simulink model "MIL4L3_SW6_V1_20220211"  (R2018b)
settings: Solver=FixedStepAuto  StartTime=0.0  StopTime=inf  FixedStep=0.001  RelTol=1e-3
PreLoadFcn:
  | A0_MILtest;
undefined symbols (not defined in the file or in its folder): Clb_ICADirect_LaneDisp_StateFive, Clb_ICADirect_LaneDisp_StateFour, Clb_ICADirect_LaneDisp_StateOne, Clb_ICADirect_LaneDisp_StateThree, Clb_ICADirect_LaneDisp_StateTwo, Clb_ICADirect_LaneDisp_StateZero, Clb_ICADirect_LaneDispSW, Clb_ICADirect_TrnLghtsCom_Switch, Clb_ICADirect_TrnLghtsCom_Value, Clb_ICADirect_TrnLghtsCrtl_Inhb, IMAP_Clb_ACU_Driver_Belt, IMAP_Clb_ACU_Driver_Belt_Over, IMAP_Clb_ACU_Passenger_Belt, IMAP_Clb_ACU_Passenger_Belt_Over, IMAP_Clb_ACU_RearLeft_Belt, IMAP_Clb_ACU_RearLeft_Belt_Over, IMAP_Clb_ACU_RearMiddle_Belt, IMAP_Clb_ACU_RearMiddle_Belt_Over, IMAP_Clb_ACU_RearRight_Belt, IMAP_Clb_ACU_RearRight_Belt_Over, IMAP_Clb_AEB_Switch, IMAP_Clb_AEB_Switch_Over, IMAP_Clb_ALC_TLC_Mode, IMAP_Clb_ALC_TLC_Mode_Over, IMAP_Clb_BCM_Battery_Voltage, IMAP_Clb_BCM_Battery_Voltage_Over, IMAP_Clb_BCM_BrakeLamp_State, IMAP_Clb_BCM_BrakeLamp_State_Over, IMAP_Clb_BCM_CHMSL_Status, IMAP_Clb_BCM_CHMSL_Status_Over, IMAP_Clb_BCM_Door_Lock_State, IMAP_Clb_BCM_Door_Lock_State_Over, IMAP_Clb_BCM_FrontWiper_State, IMAP_Clb_BCM_FrontWiper_State_Over, IMAP_Clb_BCM_FrontWiper_Switch, IMAP_Clb_BCM_FrontWiper_Switch_Over, IMAP_Clb_BCM_HazardLamp, IMAP_Clb_BCM_HazardLamp_Over, IMAP_Clb_BCM_HazardLamp_Switch, IMAP_Clb_BCM_HazardLamp_Switch_Over, IMAP_Clb_BCM_HighBeam_State, IMAP_Clb_BCM_HighBeam_State_Over, IMAP_Clb_BCM_Ignition_State, IMAP_Clb_BCM_Ignition_State_Over, IMAP_Clb_BCM_IHBC_Enabled, IMAP_Clb_BCM_IHBC_Enabled_Over, IMAP_Clb_BCM_Left_Light, IMAP_Clb_BCM_Left_Light_Over, IMAP_Clb_BCM_LeftTurn_Switch, IMAP_Clb_BCM_LeftTurn_Switch_Over, IMAP_Clb_BCM_LF_Door_State, IMAP_Clb_BCM_LF_Door_State_Over, IMAP_Clb_BCM_LowBeam_State, IMAP_Clb_BCM_LowBeam_State_Over, IMAP_Clb_BCM_LR_Door_State, IMAP_Clb_BCM_LR_Door_State_Over, IMAP_Clb_BCM_RF_Door_State, IMAP_Clb_BCM_RF_Door_State_Over, IMAP_Clb_BCM_Right_Light, IMAP_Clb_BCM_Right_Light_Over ... (+547)
libraries: CarMaker4SL x2153, simulink x292, dspstat3 x3, canmsglib x2, simulink_extras x1
(part 8 of 52)

== system MIL4L3_SW6_V1_20220211/CarMaker/VehicleControl/Function/ACC ==
  Bus Selector : BusSelector  OutputSignals=IMAPve_d_ISA_Switch,IMAPve_d_ISA_ISLC_Mode,IMAPve_d_Speed_Limit,IMAPve_d_ALC_TLC_Mode,IMAPve_d_EPS_LKA_State,IMAPve_g_EPS_SW_Trq,IMAPve_d_EPS_Trq_State,IMAPve_d_SAS_Clb_State,IMAPve_d_SAS_Trim_State,IMAPve_d_EPS_TrqLim_State,IMAPve_g_EPS_LKA_Current,IMAPve_g_ESC_LatAcc,IMAPve_d_ESC_LatAcc_Valid,IMAPve_g_ESC_YawRate,IMAPve_d_ESC_YawRate_Valid,IMAPve_g_ESC_UnYawRate,IMAPve_g_ESC_VehSpd,IMAPve_g_ESC_LonAcc,IMAPve_d_ESC_LonAcc_Valid,IMAPve_g_ESC_Brake_Press,IMAPve_g_ESC_Static_Slope,IMAPve_g_ESC_DySlope_Accuracy,IMAPve_g_ESC_DySlope,IMAPve_g_SW_Angle,IMAPve_g_SW_Angle_Speed,IMAPve_d_BCM_HazardLamp,IMAPve_d_BCM_Left_Light,IMAPve_d_BCM_Right_Light,IMAPve_d_ESC_BrakeLamp_Req,IMAPve_d_BCM_Opening_State,IMAPve_d_BCM_Trunk_State,IMAPve_d_BCM_LF_Door_State,IMAPve_d_BCM_RF_Door_State,IMAPve_d_BCM_RR_Door_State,IMAPve_d_BCM_LR_Door_State,IMAPve_d_SCC_Left_SwitchSig,IMAPve_d_SCC_Right_SwitchSig,IMAPve_d_EMS_ACC_Status,IMAPve_g_EMS_Pot_WhlT_Max,IMAPve_g_EMS_Pot_WhlT_Min,IMAPve_g_EMS_RealPedal,IMAPve_g_EMS_MaxTWhl,IMAPve_g_EMS_MaxTWhl_Offset,IMAPve_g_EMS_MinTWhl,IMAPve_g_EMS_MinTWhl_Offset,IMAPve_g_EMS_Actual_FlwT,IMAPve_g_EMS_Actual_IndT,IMAPve_g_EMS_Realize_TWhl,IMAPve_g_EMS_ACC_VirtualPedal,IMAPve_d_EMS_AccPedal_Fault,IMAPve_g_EMS_Driver_Torque,IMAPve_d_ESC_Brake_Effort,IMAPve_g_EMS_Engine_Speed,IMAPve_d_ESC_Veh_Standstill,IMAPve_d_TCU_Actual_Gear,IMAPve_d_TCU_Target_Gear,IMAPve_d_TCU_PRND_State,IMAPve_d_BCM_Ignition_State,IMAPve_d_ACU_Driver_Belt,IMAPve_d_SWS_Failure_Status,IMAPve_d_ESC_OFF,IMAPve_d_ESC_AlarmSig,IMAPve_d_ESC_ESC_Active,IMAPve_d_ESC_MSR_Active,IMAPve_d_ESC_TCS_Active,IMAPve_d_ESC_VehSpd_Valid,IMAPve_d_ESC_ABS_Active,IMAPve_d_ESC_ABS_Valid,IMAPve_d_ESC_ABS_AlarmSig,IMAPve_d_ESC_FL_WheelPulVal,IMAPve_d_ESC_FR_WheelPulVal,IMAPve_d_ESC_RL_WheelPulVal,IMAPve_d_ESC_RR_WheelPulVal,IMAPve_g_ESC_FL_WhlSpd,IMAPve_d_ESC_FL_WhlSpd_Fault,IMAPve_g_ESC_FR_WhlSpd,IMAPve_d_ESC_FR_WhlSpd_Fault,IMAPve_g_ESC_RL_WhlSpd,IMAPve_d_ESC_RL_WhlSpd_Fault,IMAPve_g_ESC_RR_WhlSpd,IMAPve_d_ESC_RR_WhlSpd_Fault,IMAPve_d_ESC_FL_Wheel_Pulse,IMAPve_d_ESC_FR_Wheel_Pulse,IMAPve_d_ESC_RL_Wheel_Pulse,IMAPve_d_ESC_RR_Wheel_Pulse,IMAPve_d_TCU_AT_Failure,IMAPve_d_TCU_Shift_Valid,IMAPve_d_TCU_DCT_Clutch_State,IMAPve_d_TCU_Gear_Engage,IMAPve_d_TCU_Select_ATMode,IMAPve_d_EMS_Engine_Status,IMAPve_d_EMS_Gearbox_CtlAvail,IMAPve_d_ESC_Brake_Failsafe,IMAPve_d_ESC_ACC_Available,IMAPve_d_ESC_ACC_Active,IMAPve_d_EMS_ACC_Effective,IMAPve_d_BCM_FrontWiper_State,IMAPve_d_BCM_CHMSL_Status,IMAPve_d_BCM_BrakeLamp_State,IMAPve_d_ACU_Passenger_Belt,IMAPve_d_EMS_ACC_CtlAvail,IMAPve_d_EMS_ACC_Inhibited,IMAPve_d_EMS_Brake_Pedal,IMAPve_d_BCM_LowBeam_State,IMAPve_d_BCM_HighBeam_State,IMAPve_d_EPB_Status,IMAPve_d_ESC_Drive_Direction,IMAPve_d_ESC_Hold_State,IMAPve_d_EPS_Steer_Hold_State,IMAPve_d_EPS_Warning_State,IMAPve_g_EPS_PowerCon,IMAPve_d_ESC_EBD_AlarmSig,IMAPve_d_ESC_AVH_Status,IMAPve_d_Radar_State,IMAPve_d_Time_System_Clock
  Bus Selector1 : BusSelector  OutputSignals=IMAPve_d_ORI_CIPV_ID,IMAPve_d_ORI_Obj_Num,IMAPva_d_ORI_Obj_Class,IMAPva_g_ORI_Obj_RelVel,IMAPva_g_ORI_Obj_LongDis,IMAPva_g_ORI_Obj_LAngle,IMAPva_g_ORI_Obj_RAngle,IMAPva_g_ORI_Obj_Width,IMAPva_d_ORI_Obj_ID,IMAPve_g_ORI_L0_C3,IMAPve_g_ORI_L0_C2,IMAPve_g_ORI_L0_C1,IMAPve_g_ORI_L0_C0,IMAPve_d_ORI_L0_Type,IMAPve_g_ORI_L0_VR,IMAPve_g_ORI_L0_W,IMAPve_g_ORI_L1_C3,IMAPve_g_ORI_L1_C2,IMAPve_g_ORI_L1_C1,IMAPve_g_ORI_L1_C0,IMAPve_d_ORI_L1_Type,IMAPve_g_ORI_L1_VR,IMAPve_g_ORI_L1_W,IMAPve_g_ORI_R0_C3,IMAPve_g_ORI_R0_C2,IMAPve_g_ORI_R0_C1,IMAPve_g_ORI_R0_C0,IMAPve_d_ORI_R0_LT,IMAPve_g_ORI_R0_VR,IMAPve_g_ORI_R0_W,IMAPve_g_ORI_R1_C3,IMAPve_g_ORI_R1_C2,IMAPve_g_ORI_R1_C1,IMAPve_g_ORI_R1_C0,IMAPve_d_ORI_R1_LT,IMAPve_g_ORI_R1_VR,IMAPve_g_ORI_R1_W,IMAPve_d_Sensor_Status,IMAPve_d_LF_Radar_Status,IMAPve_d_RF_Radar_Status,IMAPve_d_LR_Radar_Status,IMAPve_d_RR_Radar_Status,IMAPve_d_Fusion_Status,IMAPve_d_Fusion_Time_Stamp,IMAPve_d_obj_Num,IMAPva_d_obj_id,IMAPva_g_obj_pos_x,IMAPva_g_obj_pos_y,IMAPva_g_obj_vel_x,IMAPva_g_obj_vel_y,IMAPva_g_obj_acc_x,IMAPva_g_obj_acc_y,IMAPva_g_obj_pos_var_x,IMAPva_g_obj_pos_var_y,IMAPva_g_obj_pos_var_xy,IMAPva_g_obj_width,IMAPva_g_obj_length,IMAPva_d_obj_class,IMAPva_d_obj_lane,IMAPva_d_obj_status,IMAPva_d_obj_age,IMAPva_d_obj_TurnLight,IMAPva_d_obj_BrakeLight,IMAPva_d_obj_MotionStatus,IMAPve_d_Road_Type,IMAPve_g_L0_C0,IMAPve_g_L0_C1,IMAPve_g_L0_C2,IMAPve_g_L0_C3,IMAPve_g_L0_VR,IMAPve_d_L0_Q,IMAPve_d_L0_Type,IMAPve_g_L0_W,IMAPve_g_R0_C0,IMAPve_g_R0_C1,IMAPve_g_R0_C2,IMAPve_g_R0_C3,IMAPve_g_R0_VR,IMAPve_d_R0_Q,IMAPve_d_R0_Type,IMAPve_g_R0_W,IMAPve_g_L1_C0,IMAPve_g_L1_C1,IMAPve_g_L1_C2,IMAPve_g_L1_C3,IMAPve_g_L1_VR,IMAPve_d_L1_Q,IMAPve_d_L1_Type,IMAPve_g_L1_W,IMAPve_g_R1_C0,IMAPve_g_R1_C1,IMAPve_g_R1_C2,IMAPve_g_R1_C3,IMAPve_g_R1_VR,IMAPve_d_R1_Q,IMAPve_d_R1_Type,IMAPve_g_R1_W,IMAPve_g_L0_C0_Back,IMAPve_g_L0_C1_Back,IMAPve_g_L0_C2_Back,IMAPve_g_L0_C3_Back,IMAPve_g_L0_Range_Back,IMAPve_g_R0_C0_Back,IMAPve_g_R0_C1_Back,IMAPve_g_R0_C2_Back,IMAPve_g_R0_C3_Back,IMAPve_g_R0_Range_Back,IMAPve_g_L1_C0_Back,IMAPve_g_L1_C1_Back,IMAPve_g_L1_C2_Back,IMAPve_g_L1_C3_Back,IMAPve_g_L1_Range_Back,IMAPve_g_R1_C0_Back,IMAPve_g_R1_C1_Back,IMAPve_g_R1_C2_Back,IMAPve_g_R1_C3_Back,IMAPve_g_R1_Range_Back,IMAPve_d_Sign_ISA_Value,IMAPve_g_Camera_Signal_Fault,IMAPve_d_Camera_State,IMAPve_d_ESC_FLW_Direction,IMAPve_d_ESC_FRW_Direction,IMAPve_d_ESC_TCS_ErrorStatus,IMAPve_d_ESC_RLW_Direction,IMAPve_d_ESC_RRW_Direction,IMAPve_d_ESC_EPB_ErrorStatus,IMAPve_d_EPS_SteeringAngle_Flag,IMAPve_g_EPS_SteeringAngle,IMAPve_d_EPS_Driver_Override,IMAPve_d_EPS_Driver_Active_ESA,IMAPve_d_EPS_ESA_State,IMAPve_d_ACU_RearLeft_Belt,IMAPve_d_ACU_RearMiddle_Belt,IMAPve_d_ACU_RearRight_Belt,IMAPve_d_EMS_PowertrainCtl_State,IMAPve_d_TCU_TCU_Available,IMAPve_d_BCM_LeftTurn_Switch,IMAPve_d_BCM_RightTurn_Switch,IMAPve_d_MP5_AutoPilot_Switch,IMAPve_d_MP5_DMS_Sensity,IMAPve_d_MP5_DMS_EyeFatigue,IMAPve_d_MP5_DMS_LongtimeDrive,IMAPve_d_MP5_DMS_SideView,IMAPve_d_MP5_DMS_UsingPhone,IMAPve_d_MP5_DMS_Smoking,IMAPve_d_MP5_DMS_DrinkWater,IMAPve_d_APA_AutoPark_WorkSt,IMAPve_g_ESC_BrkWhlCylinder_Pressure,IMAPve_d_ISA_Status,IMAPve_d_ISA_Sign_Type,IMAPve_d_ISA_Popup_Message
  Bus Selector2 : BusSelector  OutputSignals=IMAPve_d_Camera_State
  Bus Selector3 : BusSelector  OutputSignals=AEBSve_d_AEBAlertReq
  Bus Selector4 : BusSelector  OutputSignals=IMAPva_g_ORI_Obj_ExistProb,IMAPve_d_Radar_FaultBitSetting_Signal
  Bus Selector5 : BusSelector  OutputSignals=IMAPve_d_BCM_HazardLamp_Switch
  BusCreator : BusCreator  Inputs=27
  Clock : Clock
  Data Type Conversion{,1..11,13,23..24} (15 alike) : DataTypeConversion
  Delay : Delay  DelayLength=1
  Model1 : ModelReference  ModelNameDialog=ACCS_SW6_20220127_Version.slxp  ModelReferenceVersion=1.4  CopyOfModelProtected=on
  tag scope: ACCSva_d_ACCS2ICAB=global, ACC_output=global, ADAS_ACC_State=global
  wires:
  Clock/1 -> Data Type Conversion/1  "TIME_System_Clock"
  Model1/1 -> [ADAS_ACC_State], BusCreator/1  "ACCSve_d_ACC_State"
  Model1/2 -> BusCreator/2  "ACCSve_g_ACC_TqReq"
  Model1/3 -> BusCreator/3  "ACCSve_d_ACC_TqFlag"
  Model1/4 -> BusCreator/4  "ACCSve_g_ACC_DecReq"
  Model1/5 -> BusCreator/5  "ACCSve_d_ACC_DecFlag"
  Model1/6 -> BusCreator/6  "ACCSve_d_CIPV_ID"
  Model1/7 -> BusCreator/7  "ACCSve_d_ACCActive_Signal"
  Model1/8 -> BusCreator/8  "ACCSve_d_ACC_go_request"
  Model1/9 -> BusCreator/9  "ACCSve_d_VelocitySet"
  Model1/10 -> BusCreator/10  "ACCSve_d_HeadWaySet"
  Model1/11 -> Delay/1, BusCreator/11  "ACCSva_d_ACCS2ICA"
  [ICABva_d_ICAB2ACCS] -> Model1/119
  [FDMMve_d_AccFcnConf] -> Model1/118
  Delay/1 -> [ACCSva_d_ACCS2ICAB]
  Data Type Conversion23/1 -> BusCreator/14  "ACCSve_d_ACC_ESCDriverOff"
  Data Type Conversion24/1 -> BusCreator/15  "ACCSve_d_ACC_ESCHoldReq"
  Data Type Conversion1/1 -> BusCreator/16  "ACCSve_d_ACC_EPBReq"
  Model1/16 -> Data Type Conversion1/1
  Model1/15 -> Data Type Conversion24/1
  Model1/14 -> Data Type Conversion23/1
  Data Type Conversion/1 -> Model1/116
  BusCreator/1 -> [ACC_output]
  Model1/17 -> Data Type Conversion2/1
  Model1/18 -> Data Type Conversion3/1
  Model1/19 -> Data Type Conversion4/1
  Model1/20 -> Data Type Conversion5/1
  Model1/21 -> Data Type Conversion6/1
  Model1/22 -> Data Type Conversion8/1
  Model1/23 -> Data Type Conversion7/1
  Model1/24 -> Data Type Conversion9/1
  Model1/25 -> Data Type Conversion10/1
  Model1/26 -> Data Type Conversion11/1
  Data Type Conversion2/1 -> BusCreator/17  "ACCSve_d_ACC_ISLCState"
  Data Type Conversion3/1 -> BusCreator/18  "ACCSve_d_ACC_ISLCDriverRemind"
  Data Type Conversion4/1 -> BusCreator/19  "ACCSve_d_ACCMessagePrompt"
  Data Type Conversion5/1 -> BusCreator/20  "ACCSve_g_ob1H_10"
  Data Type Conversion6/1 -> BusCreator/21  "ACCSve_g_ob1L_10"
  Data Type Conversion8/1 -> BusCreator/22  "ACCSve_g_ob2H_10"
  Data Type Conversion7/1 -> BusCreator/23  "ACCSve_g_ob2L_10"
  Data Type Conversion9/1 -> BusCreator/24  "ACCSve_g_ob01H_100"
  Data Type Conversion10/1 -> BusCreator/25  "ACCSve_g_ob01L_100"
  Data Type Conversion11/1 -> BusCreator/26  "ACCSve_g_ob02H_100"
  [AEBSve_d_MDDdecRequest] -> Model1/117
  Model1/12 -> BusCreator/12  "ACCSve_d_SignalTStamp"
  Model1/13 -> BusCreator/13  "ACCSve_d_ACC_ICA_Flag"
  Model1/27 -> Data Type Conversion13/1  "ACCSve_g_ob02L_100"
  Data Type Conversion13/1 -> BusCreator/27  "ACCSve_g_ob02L_100"
  [IMAP_Output] -> Bus Selector5/1, Bus Selector4/1, Bus Selector2/1, Bus Selector1/1, Bus Selector/1
  Bus Selector/5 -> Model1/5  "<IMAPve_d_EPS_LKA_State>"
  [AEB_output] -> Bus Selector3/1
  Bus Selector3/1 -> Model1/271  "<AEBSve_d_AEBAlertReq>"
  Bus Selector2/1 -> Model1/272  "<IMAPve_d_Camera_State>"
  Bus Selector/1 -> Model1/1  "<IMAPve_d_ISA_Switch>"
  Bus Selector/2 -> Model1/2  "<IMAPve_d_ISA_ISLC_Mode>"
  Bus Selector/3 -> Model1/3  "<IMAPve_d_Speed_Limit>"
  Bus Selector/4 -> Model1/4  "<IMAPve_d_ALC_TLC_Mode>"
  Bus Selector/6 -> Model1/6  "<IMAPve_g_EPS_SW_Trq>"
  Bus Selector/7 -> Model1/7  "<IMAPve_d_EPS_Trq_State>"
  Bus Selector/8 -> Model1/8  "<IMAPve_d_SAS_Clb_State>"
  Bus Selector/9 -> Model1/9  "<IMAPve_d_SAS_Trim_State>"
  Bus Selector/10 -> Model1/10  "<IMAPve_d_EPS_TrqLim_State>"
  Bus Selector/11 -> Model1/11  "<IMAPve_g_EPS_LKA_Current>"
  Bus Selector/12 -> Model1/12  "<IMAPve_g_ESC_LatAcc>"
  Bus Selector/13 -> Model1/13  "<IMAPve_d_ESC_LatAcc_Valid>"
  Bus Selector/14 -> Model1/14  "<IMAPve_g_ESC_YawRate>"
  Bus Selector/15 -> Model1/15  "<IMAPve_d_ESC_YawRate_Valid>"
  Bus Selector/16 -> Model1/16  "<IMAPve_g_ESC_UnYawRate>"
  Bus Selector/17 -> Model1/17  "<IMAPve_g_ESC_VehSpd>"
  Bus Selector/18 -> Model1/18  "<IMAPve_g_ESC_LonAcc>"
  Bus Selector/19 -> Model1/19  "<IMAPve_d_ESC_LonAcc_Valid>"
  Bus Selector/20 -> Model1/20  "<IMAPve_g_ESC_Brake_Press>"
  Bus Selector/21 -> Model1/21  "<IMAPve_g_ESC_Static_Slope>"
  Bus Selector/22 -> Model1/22  "<IMAPve_g_ESC_DySlope_Accuracy>"
  Bus Selector/23 -> Model1/23  "<IMAPve_g_ESC_DySlope>"
  Bus Selector/24 -> Model1/24  "<IMAPve_g_SW_Angle>"
  Bus Selector/25 -> Model1/25  "<IMAPve_g_SW_Angle_Speed>"
  Bus Selector/26 -> Model1/26  "<IMAPve_d_BCM_HazardLamp>"
  Bus Selector/27 -> Model1/27  "<IMAPve_d_BCM_Left_Light>"
  Bus Selector/28 -> Model1/28  "<IMAPve_d_BCM_Right_Light>"
  Bus Selector/29 -> Model1/29  "<IMAPve_d_ESC_BrakeLamp_Req>"
  Bus Selector/30 -> Model1/30  "<IMAPve_d_BCM_Opening_State>"
  Bus Selector/31 -> Model1/31  "<IMAPve_d_BCM_Trunk_State>"
  Bus Selector/32 -> Model1/32  "<IMAPve_d_BCM_LF_Door_State>"
  Bus Selector/33 -> Model1/33  "<IMAPve_d_BCM_RF_Door_State>"
  Bus Selector/34 -> Model1/34  "<IMAPve_d_BCM_RR_Door_State>"
  Bus Selector/35 -> Model1/35  "<IMAPve_d_BCM_LR_Door_State>"
  Bus Selector/36 -> Model1/36  "<IMAPve_d_SCC_Left_SwitchSig>"
  Bus Selector/37 -> Model1/37  "<IMAPve_d_SCC_Right_SwitchSig>"
  Bus Selector/38 -> Model1/38  "<IMAPve_d_EMS_ACC_Status>"
  Bus Selector/39 -> Model1/39  "<IMAPve_g_EMS_Pot_WhlT_Max>"
  Bus Selector/40 -> Model1/40  "<IMAPve_g_EMS_Pot_WhlT_Min>"
  Bus Selector/41 -> Model1/41  "<IMAPve_g_EMS_RealPedal>"
  Bus Selector/42 -> Model1/42  "<IMAPve_g_EMS_MaxTWhl>"
  Bus Selector/43 -> Model1/43  "<IMAPve_g_EMS_MaxTWhl_Offset>"
  Bus Selector/44 -> Model1/44  "<IMAPve_g_EMS_MinTWhl>"
  Bus Selector/45 -> Model1/45  "<IMAPve_g_EMS_MinTWhl_Offset>"
  Bus Selector/46 -> Model1/46  "<IMAPve_g_EMS_Actual_FlwT>"
  Bus Selector/47 -> Model1/47  "<IMAPve_g_EMS_Actual_IndT>"
  Bus Selector/48 -> Model1/48  "<IMAPve_g_EMS_Realize_TWhl>"
  Bus Selector/49 -> Model1/49  "<IMAPve_g_EMS_ACC_VirtualPedal>"
  Bus Selector/50 -> Model1/50  "<IMAPve_d_EMS_AccPedal_Fault>"
  Bus Selector/51 -> Model1/51  "<IMAPve_g_EMS_Driver_Torque>"
  Bus Selector/52 -> Model1/52  "<IMAPve_d_ESC_Brake_Effort>"
  Bus Selector/53 -> Model1/53  "<IMAPve_g_EMS_Engine_Speed>"
  Bus Selector/54 -> Model1/54  "<IMAPve_d_ESC_Veh_Standstill>"
  Bus Selector/55 -> Model1/55  "<IMAPve_d_TCU_Actual_Gear>"
  Bus Selector/56 -> Model1/56  "<IMAPve_d_TCU_Target_Gear>"
  Bus Selector/57 -> Model1/57  "<IMAPve_d_TCU_PRND_State>"
  Bus Selector/58 -> Model1/58  "<IMAPve_d_BCM_Ignition_State>"
  Bus Selector/59 -> Model1/59  "<IMAPve_d_ACU_Driver_Belt>"
  Bus Selector/60 -> Model1/60  "<IMAPve_d_SWS_Failure_Status>"
  Bus Selector/61 -> Model1/61  "<IMAPve_d_ESC_OFF>"
  Bus Selector/62 -> Model1/62  "<IMAPve_d_ESC_AlarmSig>"
  Bus Selector/63 -> Model1/63  "<IMAPve_d_ESC_ESC_Active>"
  Bus Selector/64 -> Model1/64  "<IMAPve_d_ESC_MSR_Active>"
  Bus Selector/65 -> Model1/65  "<IMAPve_d_ESC_TCS_Active>"
  Bus Selector/66 -> Model1/66  "<IMAPve_d_ESC_VehSpd_Valid>"
  Bus Selector/67 -> Model1/67  "<IMAPve_d_ESC_ABS_Active>"
  Bus Selector/68 -> Model1/68  "<IMAPve_d_ESC_ABS_Valid>"
  Bus Selector/69 -> Model1/69  "<IMAPve_d_ESC_ABS_AlarmSig>"
  Bus Selector/70 -> Model1/70  "<IMAPve_d_ESC_FL_WheelPulVal>"
  Bus Selector/71 -> Model1/71  "<IMAPve_d_ESC_FR_WheelPulVal>"
  Bus Selector/72 -> Model1/72  "<IMAPve_d_ESC_RL_WheelPulVal>"
  Bus Selector/73 -> Model1/73  "<IMAPve_d_ESC_RR_WheelPulVal>"
  Bus Selector/74 -> Model1/74  "<IMAPve_g_ESC_FL_WhlSpd>"
  Bus Selector/75 -> Model1/75  "<IMAPve_d_ESC_FL_WhlSpd_Fault>"
  Bus Selector/76 -> Model1/76  "<IMAPve_g_ESC_FR_WhlSpd>"
  Bus Selector/77 -> Model1/77  "<IMAPve_d_ESC_FR_WhlSpd_Fault>"
  Bus Selector/78 -> Model1/78  "<IMAPve_g_ESC_RL_WhlSpd>"
  Bus Selector/79 -> Model1/79  "<IMAPve_d_ESC_RL_WhlSpd_Fault>"
  Bus Selector/80 -> Model1/80  "<IMAPve_g_ESC_RR_WhlSpd>"
  Bus Selector/81 -> Model1/81  "<IMAPve_d_ESC_RR_WhlSpd_Fault>"
  Bus Selector/82 -> Model1/82  "<IMAPve_d_ESC_FL_Wheel_Pulse>"
  Bus Selector/83 -> Model1/83  "<IMAPve_d_ESC_FR_Wheel_Pulse>"
  Bus Selector/84 -> Model1/84  "<IMAPve_d_ESC_RL_Wheel_Pulse>"
  Bus Selector/85 -> Model1/85  "<IMAPve_d_ESC_RR_Wheel_Pulse>"
  Bus Selector/86 -> Model1/86  "<IMAPve_d_TCU_AT_Failure>"
  Bus Selector/87 -> Model1/87  "<IMAPve_d_TCU_Shift_Valid>"
  Bus Selector/88 -> Model1/88  "<IMAPve_d_TCU_DCT_Clutch_State>"
  Bus Selector/89 -> Model1/89  "<IMAPve_d_TCU_Gear_Engage>"
  Bus Selector/90 -> Model1/90  "<IMAPve_d_TCU_Select_ATMode>"
  Bus Selector/91 -> Model1/91  "<IMAPve_d_EMS_Engine_Status>"
  Bus Selector/92 -> Model1/92  "<IMAPve_d_EMS_Gearbox_CtlAvail>"
  Bus Selector/93 -> Model1/93  "<IMAPve_d_ESC_Brake_Failsafe>"
  Bus Selector/94 -> Model1/94  "<IMAPve_d_ESC_ACC_Available>"
  Bus Selector/95 -> Model1/95  "<IMAPve_d_ESC_ACC_Active>"
  Bus Selector/96 -> Model1/96  "<IMAPve_d_EMS_ACC_Effective>"
  Bus Selector/97 -> Model1/97  "<IMAPve_d_BCM_FrontWiper_State>"
  Bus Selector/98 -> Model1/98  "<IMAPve_d_BCM_CHMSL_Status>"
  Bus Selector/99 -> Model1/99  "<IMAPve_d_BCM_BrakeLamp_State>"
  Bus Selector/100 -> Model1/100  "<IMAPve_d_ACU_Passenger_Belt>"
  Bus Selector/101 -> Model1/101  "<IMAPve_d_EMS_ACC_CtlAvail>"
  Bus Selector/102 -> Model1/102  "<IMAPve_d_EMS_ACC_Inhibited>"
  Bus Selector/103 -> Model1/103  "<IMAPve_d_EMS_Brake_Pedal>"
  Bus Selector/104 -> Model1/104  "<IMAPve_d_BCM_LowBeam_State>"
  Bus Selector/105 -> Model1/105  "<IMAPve_d_BCM_HighBeam_State>"
  Bus Selector/106 -> Model1/106  "<IMAPve_d_EPB_Status>"
  Bus Selector/107 -> Model1/107  "<IMAPve_d_ESC_Drive_Direction>"
  Bus Selector/108 -> Model1/108  "<IMAPve_d_ESC_Hold_State>"
  Bus Selector/109 -> Model1/109  "<IMAPve_d_EPS_Steer_Hold_State>"
  Bus Selector/110 -> Model1/110  "<IMAPve_d_EPS_Warning_State>"
  Bus Selector/111 -> Model1/111  "<IMAPve_g_EPS_PowerCon>"
  Bus Selector/112 -> Model1/112  "<IMAPve_d_ESC_EBD_AlarmSig>"
  Bus Selector/113 -> Model1/113  "<IMAPve_d_ESC_AVH_Status>"
  Bus Selector/114 -> Model1/114  "<IMAPve_d_Radar_State>"
  Bus Selector/115 -> Model1/115  "<IMAPve_d_Time_System_Clock>"
  Bus Selector1/1 -> Model1/120  "<IMAPve_d_ORI_CIPV_ID>"
  Bus Selector1/2 -> Model1/121  "<IMAPve_d_ORI_Obj_Num>"
  Bus Selector1/3 -> Model1/122  "<IMAPva_d_ORI_Obj_Class>"
  Bus Selector1/4 -> Model1/123  "<IMAPva_g_ORI_Obj_RelVel>"
  Bus Selector1/5 -> Model1/124  "<IMAPva_g_ORI_Obj_LongDis>"
  Bus Selector1/6 -> Model1/125  "<IMAPva_g_ORI_Obj_LAngle>"
  Bus Selector1/7 -> Model1/126  "<IMAPva_g_ORI_Obj_RAngle>"
  Bus Selector1/8 -> Model1/127  "<IMAPva_g_ORI_Obj_Width>"
  Bus Selector1/9 -> Model1/128  "<IMAPva_d_ORI_Obj_ID>"
  Bus Selector1/10 -> Model1/129  "<IMAPve_g_ORI_L0_C3>"
  Bus Selector1/11 -> Model1/130  "<IMAPve_g_ORI_L0_C2>"
  Bus Selector1/12 -> Model1/131  "<IMAPve_g_ORI_L0_C1>"
  Bus Selector1/13 -> Model1/132  "<IMAPve_g_ORI_L0_C0>"
  Bus Selector1/14 -> Model1/133  "<IMAPve_d_ORI_L0_Type>"
  Bus Selector1/15 -> Model1/134  "<IMAPve_g_ORI_L0_VR>"
  Bus Selector1/16 -> Model1/135  "<IMAPve_g_ORI_L0_W>"
  Bus Selector1/17 -> Model1/136  "<IMAPve_g_ORI_L1_C3>"
  Bus Selector1/18 -> Model1/137  "<IMAPve_g_ORI_L1_C2>"
  Bus Selector1/19 -> Model1/138  "<IMAPve_g_ORI_L1_C1>"
  Bus Selector1/20 -> Model1/139  "<IMAPve_g_ORI_L1_C0>"
  Bus Selector1/21 -> Model1/140  "<IMAPve_d_ORI_L1_Type>"
  Bus Selector1/22 -> Model1/141  "<IMAPve_g_ORI_L1_VR>"
  Bus Selector1/23 -> Model1/142  "<IMAPve_g_ORI_L1_W>"
  Bus Selector1/24 -> Model1/143  "<IMAPve_g_ORI_R0_C3>"
  Bus Selector1/25 -> Model1/144  "<IMAPve_g_ORI_R0_C2>"
  Bus Selector1/26 -> Model1/145  "<IMAPve_g_ORI_R0_C1>"
  Bus Selector1/27 -> Model1/146  "<IMAPve_g_ORI_R0_C0>"
  Bus Selector1/28 -> Model1/147  "<IMAPve_d_ORI_R0_LT>"
  Bus Selector1/29 -> Model1/148  "<IMAPve_g_ORI_R0_VR>"
  Bus Selector1/30 -> Model1/149  "<IMAPve_g_ORI_R0_W>"
  Bus Selector1/31 -> Model1/150  "<IMAPve_g_ORI_R1_C3>"
  Bus Selector1/32 -> Model1/151  "<IMAPve_g_ORI_R1_C2>"
  Bus Selector1/33 -> Model1/152  "<IMAPve_g_ORI_R1_C1>"
  Bus Selector1/34 -> Model1/153  "<IMAPve_g_ORI_R1_C0>"
  Bus Selector1/35 -> Model1/154  "<IMAPve_d_ORI_R1_LT>"
  Bus Selector1/36 -> Model1/155  "<IMAPve_g_ORI_R1_VR>"
  Bus Selector1/37 -> Model1/156  "<IMAPve_g_ORI_R1_W>"
  Bus Selector1/38 -> Model1/157  "<IMAPve_d_Sensor_Status>"
  Bus Selector1/39 -> Model1/158  "<IMAPve_d_LF_Radar_Status>"
  Bus Selector1/40 -> Model1/159  "<IMAPve_d_RF_Radar_Status>"
  Bus Selector1/41 -> Model1/160  "<IMAPve_d_LR_Radar_Status>"
  Bus Selector1/42 -> Model1/161  "<IMAPve_d_RR_Radar_Status>"
  Bus Selector1/43 -> Model1/162  "<IMAPve_d_Fusion_Status>"
  Bus Selector1/44 -> Model1/163  "<IMAPve_d_Fusion_Time_Stamp>"
  Bus Selector1/45 -> Model1/164  "<IMAPve_d_obj_Num>"
  Bus Selector1/46 -> Model1/165  "<IMAPva_d_obj_id>"
  Bus Selector1/47 -> Model1/166  "<IMAPva_g_obj_pos_x>"
  Bus Selector1/48 -> Model1/167  "<IMAPva_g_obj_pos_y>"
  Bus Selector1/49 -> Model1/168  "<IMAPva_g_obj_vel_x>"
  Bus Selector1/50 -> Model1/169  "<IMAPva_g_obj_vel_y>"
  Bus Selector1/51 -> Model1/170  "<IMAPva_g_obj_acc_x>"
  Bus Selector1/52 -> Model1/171  "<IMAPva_g_obj_acc_y>"
  Bus Selector1/53 -> Model1/172  "<IMAPva_g_obj_pos_var_x>"
  Bus Selector1/54 -> Model1/173  "<IMAPva_g_obj_pos_var_y>"
  Bus Selector1/55 -> Model1/174  "<IMAPva_g_obj_pos_var_xy>"
  Bus Selector1/56 -> Model1/175  "<IMAPva_g_obj_width>"
  Bus Selector1/57 -> Model1/176  "<IMAPva_g_obj_length>"
  Bus Selector1/58 -> Model1/177  "<IMAPva_d_obj_class>"
  Bus Selector1/59 -> Model1/178  "<IMAPva_d_obj_lane>"
  Bus Selector1/60 -> Model1/179  "<IMAPva_d_obj_status>"
  Bus Selector1/61 -> Model1/180  "<IMAPva_d_obj_age>"
  Bus Selector1/62 -> Model1/181  "<IMAPva_d_obj_TurnLight>"
  Bus Selector1/63 -> Model1/182  "<IMAPva_d_obj_BrakeLight>"
  Bus Selector1/64 -> Model1/183  "<IMAPva_d_obj_MotionStatus>"
  Bus Selector1/65 -> Model1/184  "<IMAPve_d_Road_Type>"
  Bus Selector1/66 -> Model1/185  "<IMAPve_g_L0_C0>"
  Bus Selector1/67 -> Model1/186  "<IMAPve_g_L0_C1>"
  Bus Selector1/68 -> Model1/187  "<IMAPve_g_L0_C2>"
  Bus Selector1/69 -> Model1/188  "<IMAPve_g_L0_C3>"
  Bus Selector1/70 -> Model1/189  "<IMAPve_g_L0_VR>"
  Bus Selector1/71 -> Model1/190  "<IMAPve_d_L0_Q>"
  Bus Selector1/72 -> Model1/191  "<IMAPve_d_L0_Type>"
  Bus Selector1/73 -> Model1/192  "<IMAPve_g_L0_W>"
  Bus Selector1/74 -> Model1/193  "<IMAPve_g_R0_C0>"
  Bus Selector1/75 -> Model1/194  "<IMAPve_g_R0_C1>"
  Bus Selector1/76 -> Model1/195  "<IMAPve_g_R0_C2>"
  Bus Selector1/77 -> Model1/196  "<IMAPve_g_R0_C3>"
  Bus Selector1/78 -> Model1/197  "<IMAPve_g_R0_VR>"
  Bus Selector1/79 -> Model1/198  "<IMAPve_d_R0_Q>"
  Bus Selector1/80 -> Model1/199  "<IMAPve_d_R0_Type>"
  Bus Selector1/81 -> Model1/200  "<IMAPve_g_R0_W>"
  Bus Selector1/82 -> Model1/201  "<IMAPve_g_L1_C0>"
  Bus Selector1/83 -> Model1/202  "<IMAPve_g_L1_C1>"
  Bus Selector1/84 -> Model1/203  "<IMAPve_g_L1_C2>"
  Bus Selector1/85 -> Model1/204  "<IMAPve_g_L1_C3>"
  Bus Selector1/86 -> Model1/205  "<IMAPve_g_L1_VR>"
  Bus Selector1/87 -> Model1/206  "<IMAPve_d_L1_Q>"
  Bus Selector1/88 -> Model1/207  "<IMAPve_d_L1_Type>"
  Bus Selector1/89 -> Model1/208  "<IMAPve_g_L1_W>"
  Bus Selector1/90 -> Model1/209  "<IMAPve_g_R1_C0>"
  Bus Selector1/91 -> Model1/210  "<IMAPve_g_R1_C1>"
  Bus Selector1/92 -> Model1/211  "<IMAPve_g_R1_C2>"
  Bus Selector1/93 -> Model1/212  "<IMAPve_g_R1_C3>"
  Bus Selector1/94 -> Model1/213  "<IMAPve_g_R1_VR>"
  Bus Selector1/95 -> Model1/214  "<IMAPve_d_R1_Q>"
  Bus Selector1/96 -> Model1/215  "<IMAPve_d_R1_Type>"
  Bus Selector1/97 -> Model1/216  "<IMAPve_g_R1_W>"
  Bus Selector1/98 -> Model1/217  "<IMAPve_g_L0_C0_Back>"
  Bus Selector1/99 -> Model1/218  "<IMAPve_g_L0_C1_Back>"
  Bus Selector1/100 -> Model1/219  "<IMAPve_g_L0_C2_Back>"
  Bus Selector1/101 -> Model1/220  "<IMAPve_g_L0_C3_Back>"
  Bus Selector1/102 -> Model1/221  "<IMAPve_g_L0_Range_Back>"
  Bus Selector1/103 -> Model1/222  "<IMAPve_g_R0_C0_Back>"
  Bus Selector1/104 -> Model1/223  "<IMAPve_g_R0_C1_Back>"
  Bus Selector1/105 -> Model1/224  "<IMAPve_g_R0_C2_Back>"
  Bus Selector1/106 -> Model1/225  "<IMAPve_g_R0_C3_Back>"
  Bus Selector1/107 -> Model1/226  "<IMAPve_g_R0_Range_Back>"
  Bus Selector1/108 -> Model1/227  "<IMAPve_g_L1_C0_Back>"
  Bus Selector1/109 -> Model1/228  "<IMAPve_g_L1_C1_Back>"
  Bus Selector1/110 -> Model1/229  "<IMAPve_g_L1_C2_Back>"
  Bus Selector1/111 -> Model1/230  "<IMAPve_g_L1_C3_Back>"
  Bus Selector1/112 -> Model1/231  "<IMAPve_g_L1_Range_Back>"
  Bus Selector1/113 -> Model1/232  "<IMAPve_g_R1_C0_Back>"
  Bus Selector1/114 -> Model1/233  "<IMAPve_g_R1_C1_Back>"
  Bus Selector1/115 -> Model1/234  "<IMAPve_g_R1_C2_Back>"
  Bus Selector1/116 -> Model1/235  "<IMAPve_g_R1_C3_Back>"
  Bus Selector1/117 -> Model1/236  "<IMAPve_g_R1_Range_Back>"
  Bus Selector1/118 -> Model1/237  "<IMAPve_d_Sign_ISA_Value>"
  Bus Selector1/119 -> Model1/238  "<IMAPve_g_Camera_Signal_Fault>"
  Bus Selector1/120 -> Model1/239  "<IMAPve_d_Camera_State>"
  Bus Selector1/121 -> Model1/240  "<IMAPve_d_ESC_FLW_Direction>"
  Bus Selector1/122 -> Model1/241  "<IMAPve_d_ESC_FRW_Direction>"
  Bus Selector1/123 -> Model1/242  "<IMAPve_d_ESC_TCS_ErrorStatus>"
  Bus Selector1/124 -> Model1/243  "<IMAPve_d_ESC_RLW_Direction>"
  Bus Selector1/125 -> Model1/244  "<IMAPve_d_ESC_RRW_Direction>"
  Bus Selector1/126 -> Model1/245  "<IMAPve_d_ESC_EPB_ErrorStatus>"
  Bus Selector1/127 -> Model1/246  "<IMAPve_d_EPS_SteeringAngle_Flag>"
  Bus Selector1/128 -> Model1/247  "<IMAPve_g_EPS_SteeringAngle>"
  Bus Selector1/129 -> Model1/248  "<IMAPve_d_EPS_Driver_Override>"
  Bus Selector1/130 -> Model1/249  "<IMAPve_d_EPS_Driver_Active_ESA>"
  Bus Selector1/131 -> Model1/250  "<IMAPve_d_EPS_ESA_State>"
  Bus Selector1/132 -> Model1/251  "<IMAPve_d_ACU_RearLeft_Belt>"
  Bus Selector1/133 -> Model1/252  "<IMAPve_d_ACU_RearMiddle_Belt>"
  Bus Selector1/134 -> Model1/253  "<IMAPve_d_ACU_RearRight_Belt>"
  Bus Selector1/135 -> Model1/254  "<IMAPve_d_EMS_PowertrainCtl_State>"
  Bus Selector1/136 -> Model1/255  "<IMAPve_d_TCU_TCU_Available>"
  Bus Selector1/137 -> Model1/256  "<IMAPve_d_BCM_LeftTurn_Switch>"
  Bus Selector1/138 -> Model1/257  "<IMAPve_d_BCM_RightTurn_Switch>"
  Bus Selector1/139 -> Model1/258  "<IMAPve_d_MP5_AutoPilot_Switch>"
  Bus Selector1/140 -> Model1/259  "<IMAPve_d_MP5_DMS_Sensity>"
  Bus Selector1/141 -> Model1/260  "<IMAPve_d_MP5_DMS_EyeFatigue>"
  Bus Selector1/142 -> Model1/261  "<IMAPve_d_MP5_DMS_LongtimeDrive>"
  Bus Selector1/143 -> Model1/262  "<IMAPve_d_MP5_DMS_SideView>"
  Bus Selector1/144 -> Model1/263  "<IMAPve_d_MP5_DMS_UsingPhone>"
  Bus Selector1/145 -> Model1/264  "<IMAPve_d_MP5_DMS_Smoking>"
  Bus Selector1/146 -> Model1/265  "<IMAPve_d_MP5_DMS_DrinkWater>"
  Bus Selector1/147 -> Model1/266  "<IMAPve_d_APA_AutoPark_WorkSt>"
  Bus Selector1/148 -> Model1/267  "<IMAPve_g_ESC_BrkWhlCylinder_Pressure>"
  Bus Selector1/149 -> Model1/268  "<IMAPve_d_ISA_Status>"
  Bus Selector1/150 -> Model1/269  "<IMAPve_d_ISA_Sign_Type>"
  Bus Selector1/151 -> Model1/270  "<IMAPve_d_ISA_Popup_Message>"
  Bus Selector4/1 -> Model1/274  "<IMAPva_g_ORI_Obj_ExistProb>"
  Bus Selector4/2 -> Model1/275  "<IMAPve_d_Radar_FaultBitSetting_Signal>"
  Bus Selector5/1 -> Model1/279  "<IMAPve_d_BCM_HazardLamp_Switch>"
  [MDD_deceleration_type] -> Model1/273

== system MIL4L3_SW6_V1_20220211/CarMaker/VehicleControl/Function/AEB ==
  Bus Selector : BusSelector  OutputSignals=IMAPve_d_ORI_CIPV_ID,IMAPve_d_ORI_Obj_Num,IMAPva_d_ORI_Obj_Class,IMAPva_g_ORI_Obj_RelVel,IMAPva_g_ORI_Obj_LongDis,IMAPva_g_ORI_Obj_LAngle,IMAPva_g_ORI_Obj_RAngle,IMAPva_g_ORI_Obj_Width,IMAPva_d_ORI_Obj_ID,IMAPve_d_ESC_ABS_Valid
  Bus Selector1 : BusSelector  OutputSignals=IMAPve_d_APA_AutoPark_WorkSt,IMAPve_d_EMS_AccPedal_Fault,IMAPve_d_Camera_State
  Bus Selector2 : BusSelector  OutputSignals=IMAPve_d_BCM_HazardLamp_Switch
  Bus Selector6 : BusSelector  OutputSignals=IMAPve_d_AEB_Switch,IMAPve_d_FCW_Switch,IMAPve_d_FCW_Sensitivity,IMAPve_g_ESC_LatAcc,IMAPve_g_ESC_YawRate,IMAPve_d_ESC_YawRate_Valid,IMAPve_g_ESC_VehSpd,IMAPve_g_ESC_LonAcc,IMAPve_d_ESC_LonAcc_Valid,IMAPve_g_ESC_Brake_Press,IMAPve_g_ESC_Static_Slope,IMAPve_g_ESC_DySlope_Accuracy,IMAPve_g_ESC_DySlope,IMAPve_g_SW_Angle,IMAPve_g_SW_Angle_Speed,IMAPve_d_BCM_Left_Light,IMAPve_d_BCM_Right_Light,IMAPve_d_BCM_Opening_State,IMAPve_g_EMS_RealPedal,IMAPve_d_ESC_Veh_Standstill,IMAPve_d_TCU_Actual_Gear,IMAPve_d_BCM_Ignition_State,IMAPve_d_ACU_Driver_Belt,IMAPve_d_SWS_Failure_Status,IMAPve_d_ESC_OFF,IMAPve_d_ESC_AlarmSig,IMAPve_d_ESC_ESC_Active,IMAPve_d_ESC_MSR_Active,IMAPve_d_ESC_TCS_Active,IMAPve_d_ESC_VehSpd_Valid,IMAPve_d_ESC_ABS_Active,IMAPve_d_ESC_FL_WheelPulVal,IMAPve_d_ESC_FR_WheelPulVal,IMAPve_d_ESC_RL_WheelPulVal,IMAPve_d_ESC_RR_WheelPulVal,IMAPve_d_TCU_AT_Failure,IMAPve_d_EMS_Engine_Status,IMAPve_d_ESC_AEB_Available,IMAPve_d_ESC_AEB_Active,IMAPve_d_BCM_FrontWiper_State,IMAPve_d_BCM_CHMSL_Status,IMAPve_d_BCM_BrakeLamp_State,IMAPve_d_ACU_Passenger_Belt,IMAPve_d_EMS_Brake_Pedal,IMAPve_d_EPB_Status,IMAPve_d_ESC_Drive_Direction,IMAPve_d_ESC_Hold_State,IMAPve_d_Radar_State,IMAPve_d_Time_System_Clock,IMAPve_d_Sensor_Status,IMAPve_d_LF_Radar_Status,IMAPve_d_RF_Radar_Status,IMAPve_d_LR_Radar_Status,IMAPve_d_RR_Radar_Status,IMAPve_d_Fusion_Status,IMAPve_d_Fusion_Time_Stamp,IMAPve_d_obj_Num,IMAPva_d_obj_id,IMAPva_g_obj_pos_x,IMAPva_g_obj_pos_y,IMAPva_g_obj_vel_x,IMAPva_g_obj_vel_y,IMAPva_g_obj_acc_x,IMAPva_g_obj_acc_y,IMAPva_g_obj_pos_var_x,IMAPva_g_obj_pos_var_y,IMAPva_g_obj_pos_var_xy,IMAPva_g_obj_width,IMAPva_g_obj_length,IMAPva_d_obj_class,IMAPva_d_obj_lane,IMAPva_d_obj_status,IMAPva_d_obj_age,IMAPva_d_obj_TurnLight,IMAPva_d_obj_BrakeLight,IMAPva_d_obj_MotionStatus,IMAPve_g_Camera_Signal_Fault,IMAPve_d_Camera_Status
  Bus Selector7 : BusSelector  OutputSignals=FDMMve_d_AebFcnConf,FDMMve_d_SignalTStamp
  Bus Selector8 : BusSelector  OutputSignals=JABSve_d_Switching,JABSve_g_DecelReq,JABSve_d_FltStatus,JABSve_d_AlertReq,JABSve_d_HapticAlarm,JABSve_d_Tips,JABSve_d_DbSignalTStamp
  BusCreator : BusCreator  Inputs=32
  Clock : Clock
  Data Type Conversion : DataTypeConversion
  Delay : Delay  Commented=on  DelayLength=1
  Function-Call Generator : simulink/Ports & Subsystems/Function-Call Generator  sample_time=0.01  numberOfIterations=1
  Model2 : ModelReference  ModelNameDialog=AEBS.slxp  ModelReferenceVersion=1.281  CopyOfModelProtected=on
  tag scope: AEBSve_d_MDDdecRequest=global, AEB_output=global
  wires:
  Model2/1 -> BusCreator/1  "AEBSve_d_Prefill_request"
  Model2/2 -> BusCreator/2  "AEBSve_d_functionFARCState"
  Model2/3 -> BusCreator/3  "AEBSve_g_DecSetpoint"
  Model2/4 -> [AEBSve_d_MDDdecRequest], BusCreator/4  "AEBSve_d_MDDdecRequest"
  Model2/5 -> BusCreator/5  "AEBSve_d_MDDdecType"
  Model2/6 -> BusCreator/6  "AEBSve_d_HapticAlarm"
  Model2/7 -> BusCreator/7  "AEBSve_d_Braking_progress"
  Model2/8 -> BusCreator/8  "AEBSve_d_AEBStatus"
  Model2/10 -> BusCreator/10  "AEBSve_d_AEBSwitchStatus"
  Model2/9 -> BusCreator/9  "AEBSve_d_FCWStatus"
  Model2/11 -> BusCreator/11  "AEBSve_d_AEBFaultStatus"
  Model2/13 -> BusCreator/13  "AEBSve_d_AEBTips"
  Model2/16 -> BusCreator/16  "AEBSve_d_JABS_SwitchStatus"
  Model2/12 -> BusCreator/12  "AEBSve_d_AEBAlertReq"
  Model2/14 -> BusCreator/14  "AEBSve_d_SignalTStamp"
  Model2/17 -> BusCreator/17  "AEBSve_d_JABS_FltStatus"
  Model2/15 -> BusCreator/15  "AEBSve_d_JABS_AlertSign"
  [IMAP_Output] -> Bus Selector/1, Bus Selector2/1, Bus Selector1/1, Bus Selector6/1
  [FDMM_output] -> Bus Selector7/1
  [JA_output] -> Bus Selector8/1
  BusCreator/1 -> [AEB_output]
  Model2/18 -> BusCreator/18  "AEBSve_d_JABS_AlertReq"
  Model2/19 -> BusCreator/19  "AEBSve_d_JABS_HapticAlarm"
  Model2/20 -> BusCreator/20  "AEBSve_d_JABS_Tips"
  Model2/21 -> BusCreator/21  "AEBSve_d_ESCDriverOff"
  Model2/22 -> BusCreator/22  "AEBSve_d_ESCHoldReq"
  Model2/23 -> BusCreator/23  "AEBSve_g_ob3H_10"
  Model2/24 -> BusCreator/24  "AEBSve_g_ob3L_10"
  Model2/25 -> BusCreator/25  "AEBSve_g_ob4H_10"
  Model2/26 -> BusCreator/26  "AEBSve_g_ob4L_10"
  Model2/27 -> BusCreator/27  "AEBSve_g_ob04H_100"
  Model2/28 -> BusCreator/28  "AEBSve_g_ob04L_100"
  Model2/29 -> BusCreator/29  "AEBSve_g_ob05H_100"
  Model2/30 -> BusCreator/30  "AEBSve_g_ob05L_100"
  Model2/31 -> BusCreator/31  "AEBSve_g_ob06H_100"
  Model2/32 -> BusCreator/32  "AEBSve_g_ob06L_100"
  Bus Selector1/3 -> Model2/102  "<IMAPve_d_Camera_State>"
  Bus Selector1/2 -> Model2/101  "<IMAPve_d_EMS_AccPedal_Fault>"
  Bus Selector1/1 -> Model2/100  "<IMAPve_d_APA_AutoPark_WorkSt>"
  [MDD_deceleration_type] -> Model2/99
  Data Type Conversion/1 -> Model2/88
  Clock/1 -> Data Type Conversion/1  "TIME_System_Clock"
  Bus Selector8/4 -> Model2/82  "<JABSve_d_AlertReq>"
  Bus Selector8/3 -> Model2/81  "<JABSve_d_FltStatus>"
  Bus Selector8/5 -> Model2/83  "<JABSve_d_HapticAlarm>"
  Bus Selector8/2 -> Model2/80  "<JABSve_g_DecelReq>"
  Bus Selector8/6 -> Model2/84  "<JABSve_d_Tips>"
  Bus Selector8/1 -> Model2/79  "<JABSve_d_Switching>"
  Bus Selector8/7 -> Model2/85  "<JABSve_d_DbSignalTStamp>"
  Bus Selector7/1 -> Model2/86  "<FDMMve_d_AebFcnConf>"
  Bus Selector7/2 -> Model2/87  "<FDMMve_d_SignalTStamp>"
  Bus Selector6/1 -> Model2/1  "<IMAPve_d_AEB_Switch>"
  Bus Selector6/2 -> Model2/2  "<IMAPve_d_FCW_Switch>"
  Bus Selector6/3 -> Model2/3  "<IMAPve_d_FCW_Sensitivity>"
  Bus Selector6/4 -> Model2/4  "<IMAPve_g_ESC_LatAcc>"
  Bus Selector6/5 -> Model2/5  "<IMAPve_g_ESC_YawRate>"
  Bus Selector6/6 -> Model2/6  "<IMAPve_d_ESC_YawRate_Valid>"
  Bus Selector6/7 -> Model2/7  "<IMAPve_g_ESC_VehSpd>"
  Bus Selector6/8 -> Model2/8  "<IMAPve_g_ESC_LonAcc>"
  Bus Selector6/9 -> Model2/9  "<IMAPve_d_ESC_LonAcc_Valid>"
  Bus Selector6/10 -> Model2/10  "<IMAPve_g_ESC_Brake_Press>"
  Bus Selector6/11 -> Model2/11  "<IMAPve_g_ESC_Static_Slope>"
  Bus Selector6/12 -> Model2/12  "<IMAPve_g_ESC_DySlope_Accuracy>"
  Bus Selector6/13 -> Model2/13  "<IMAPve_g_ESC_DySlope>"
  Bus Selector6/14 -> Model2/14  "<IMAPve_g_SW_Angle>"
  Bus Selector6/15 -> Model2/15  "<IMAPve_g_SW_Angle_Speed>"
  Bus Selector6/16 -> Model2/16  "<IMAPve_d_BCM_Left_Light>"
  Bus Selector6/17 -> Model2/17  "<IMAPve_d_BCM_Right_Light>"
  Bus Selector6/18 -> Model2/18  "<IMAPve_d_BCM_Opening_State>"
  Bus Selector6/19 -> Model2/19  "<IMAPve_g_EMS_RealPedal>"
  Bus Selector6/20 -> Model2/20  "<IMAPve_d_ESC_Veh_Standstill>"
  Bus Selector6/21 -> Model2/21  "<IMAPve_d_TCU_Actual_Gear>"
  Bus Selector6/22 -> Model2/22  "<IMAPve_d_BCM_Ignition_State>"
  Bus Selector6/23 -> Model2/23  "<IMAPve_d_ACU_Driver_Belt>"
  Bus Selector6/24 -> Model2/24  "<IMAPve_d_SWS_Failure_Status>"
  Bus Selector6/25 -> Model2/25  "<IMAPve_d_ESC_OFF>"
  Bus Selector6/26 -> Model2/26  "<IMAPve_d_ESC_AlarmSig>"
  Bus Selector6/27 -> Model2/27  "<IMAPve_d_ESC_ESC_Active>"
  Bus Selector6/28 -> Model2/28  "<IMAPve_d_ESC_MSR_Active>"
  Bus Selector6/29 -> Model2/29  "<IMAPve_d_ESC_TCS_Active>"
  Bus Selector6/30 -> Model2/30  "<IMAPve_d_ESC_VehSpd_Valid>"
  Bus Selector6/31 -> Model2/31  "<IMAPve_d_ESC_ABS_Active>"
  Bus Selector6/32 -> Model2/32  "<IMAPve_d_ESC_FL_WheelPulVal>"
  Bus Selector6/33 -> Model2/33  "<IMAPve_d_ESC_FR_WheelPulVal>"
  Bus Selector6/34 -> Model2/34  "<IMAPve_d_ESC_RL_WheelPulVal>"
  Bus Selector6/35 -> Model2/35  "<IMAPve_d_ESC_RR_WheelPulVal>"
  Bus Selector6/36 -> Model2/36  "<IMAPve_d_TCU_AT_Failure>"
  Bus Selector6/37 -> Model2/37  "<IMAPve_d_EMS_Engine_Status>"
  Bus Selector6/38 -> Model2/38  "<IMAPve_d_ESC_AEB_Available>"
  Bus Selector6/39 -> Model2/39  "<IMAPve_d_ESC_AEB_Active>"
  Bus Selector6/40 -> Model2/40  "<IMAPve_d_BCM_FrontWiper_State>"
  Bus Selector6/41 -> Model2/41  "<IMAPve_d_BCM_CHMSL_Status>"
  Bus Selector6/42 -> Model2/42  "<IMAPve_d_BCM_BrakeLamp_State>"
  Bus Selector6/43 -> Model2/43  "<IMAPve_d_ACU_Passenger_Belt>"
  Bus Selector6/44 -> Model2/44  "<IMAPve_d_EMS_Brake_Pedal>"
  Bus Selector6/45 -> Model2/45  "<IMAPve_d_EPB_Status>"
  Bus Selector6/46 -> Model2/46  "<IMAPve_d_ESC_Drive_Direction>"
  Bus Selector6/47 -> Model2/47  "<IMAPve_d_ESC_Hold_State>"
  Bus Selector6/48 -> Model2/48  "<IMAPve_d_Radar_State>"
  Bus Selector6/49 -> Model2/49  "<IMAPve_d_Time_System_Clock>"
  Bus Selector6/50 -> Model2/50  "<IMAPve_d_Sensor_Status>"
  Bus Selector6/51 -> Model2/51  "<IMAPve_d_LF_Radar_Status>"
  Bus Selector6/52 -> Model2/52  "<IMAPve_d_RF_Radar_Status>"
  Bus Selector6/53 -> Model2/53  "<IMAPve_d_LR_Radar_Status>"
  Bus Selector6/54 -> Model2/54  "<IMAPve_d_RR_Radar_Status>"
  Bus Selector6/55 -> Model2/55  "<IMAPve_d_Fusion_Status>"
  Bus Selector6/56 -> Model2/56  "<IMAPve_d_Fusion_Time_Stamp>"
  Bus Selector6/57 -> Model2/57  "<IMAPve_d_obj_Num>"
  Bus Selector6/58 -> Model2/58  "<IMAPva_d_obj_id>"
  Bus Selector6/59 -> Model2/59  "<IMAPva_g_obj_pos_x>"
  Bus Selector6/60 -> Model2/60  "<IMAPva_g_obj_pos_y>"
  Bus Selector6/61 -> Model2/61  "<IMAPva_g_obj_vel_x>"
  Bus Selector6/62 -> Model2/62  "<IMAPva_g_obj_vel_y>"
  Bus Selector6/63 -> Model2/63  "<IMAPva_g_obj_acc_x>"
  Bus Selector6/64 -> Model2/64  "<IMAPva_g_obj_acc_y>"
  Bus Selector6/65 -> Model2/65  "<IMAPva_g_obj_pos_var_x>"
  Bus Selector6/66 -> Model2/66  "<IMAPva_g_obj_pos_var_y>"
  Bus Selector6/67 -> Model2/67  "<IMAPva_g_obj_pos_var_xy>"
  Bus Selector6/68 -> Model2/68  "<IMAPva_g_obj_width>"
  Bus Selector6/69 -> Model2/69  "<IMAPva_g_obj_length>"
  Bus Selector6/70 -> Model2/70  "<IMAPva_d_obj_class>"
  Bus Selector6/71 -> Model2/71  "<IMAPva_d_obj_lane>"
  Bus Selector6/72 -> Model2/72  "<IMAPva_d_obj_status>"
  Bus Selector6/73 -> Model2/73  "<IMAPva_d_obj_age>"
  Bus Selector6/74 -> Model2/74  "<IMAPva_d_obj_TurnLight>"
  Bus Selector6/75 -> Model2/75  "<IMAPva_d_obj_BrakeLight>"
  Bus Selector6/76 -> Model2/76  "<IMAPva_d_obj_MotionStatus>"
  Bus Selector6/77 -> Model2/77  "<IMAPve_g_Camera_Signal_Fault>"
  Bus Selector6/78 -> Model2/78  "<IMAPve_d_Camera_Status>"
  Bus Selector/1 -> Model2/89  "<IMAPve_d_ORI_CIPV_ID>"
  Bus Selector/2 -> Model2/90  "<IMAPve_d_ORI_Obj_Num>"
  Bus Selector/3 -> Model2/91  "<IMAPva_d_ORI_Obj_Class>"
  Bus Selector/4 -> Model2/92  "<IMAPva_g_ORI_Obj_RelVel>"
  Bus Selector/5 -> Model2/93  "<IMAPva_g_ORI_Obj_LongDis>"
  Bus Selector/6 -> Model2/94  "<IMAPva_g_ORI_Obj_LAngle>"
  Bus Selector/7 -> Model2/95  "<IMAPva_g_ORI_Obj_RAngle>"
  Bus Selector/8 -> Model2/96  "<IMAPva_g_ORI_Obj_Width>"
  Bus Selector/9 -> Model2/97  "<IMAPva_d_ORI_Obj_ID>"
  Bus Selector/10 -> Model2/98  "<IMAPve_d_ESC_ABS_Valid>"
  Bus Selector2/1 -> Model2/106  "<IMAPve_d_BCM_HazardLamp_Switch>"
  Function-Call Generator/1 -> Model2/107
